simulink model "VCU_SW_1"  (R2023b)
settings: Solver=FixedStepDiscrete  StartTime=0.0  StopTime=inf  FixedStep=1e-2  RelTol=1e-3
PreLoadFcn:
  | RTWConfigurationCB('preloadfcn', bdroot);
InitFcn:
  | loadvar_ttc500
undefined symbols (not defined in the file): BrkPedalTypes, CabMovModeTypes, cFuseTempSensAcc_X, cFuseTempSensAcc_Y, cFuseTempSensVal_X, cFuseTempSensVal_Y, cTMSTempSensVal_X, cTMSTempSensVal_Y, cTransferCaseSpeedRatio, diag_state, DoorsPositionTypes, dP_filter_Y, DriverOccClassSystemTypes, ErrorValueTypes, fatal_error_callback, IO_ADC_NO_RANGE, LadderStatusTypes, pAnalogCabRotSensAcc, pAnalogCabRotSensMaxVolt, pAnalogCabRotSensMinVolt, pAnalogCabRotSensRange, pAnalogCabRotSensZeroVolt, pBrkActivePress, pCabTiltSensAcc, pCabTiltSensMaxCur, pCabTiltSensMinCur, pDistanceCorrection, pECANManual_BPNEnable, pECANManual_BPNEnabler_Flag, pFilterSensAccRes, pHDirMaxDiffFrq, pHDirSensHighLvl, pHDirSensLowLvl, pMainGearRatio, pMaxFilterSensRes, pMaxFirstPedalSensValue, pMaxFuseTempSensRes, pMaxPressLoss, pMaxPressSensCurrent, pMaxPressValue, pMaxPressValueHydMotAndPump, pMaxPressValueParkDrain, pMaxSecondPedalSensValue, pMaxTempSensVoltage, pMaxTempValue, pMaxTMSTempSensRes, pMinFilterSensRes, pMinFirstPedalSensValue, pMinFuseTempSensRes, pMinPressLoss, pMinPressSensCurrent, pMinPressValue, pMinSecondPedalSensValue, pMinTempSensVoltage, pMinTempValue, pMinTMSTempSensRes, pMotorRingTeethNum, pPedalSensAccuracyPct, pPedalSensAccuracyVolt, pPressLossTreshhold ... (+20)
libraries: TTlibrary x270, canmsglib x127, simulink x88
(part 7 of 19)

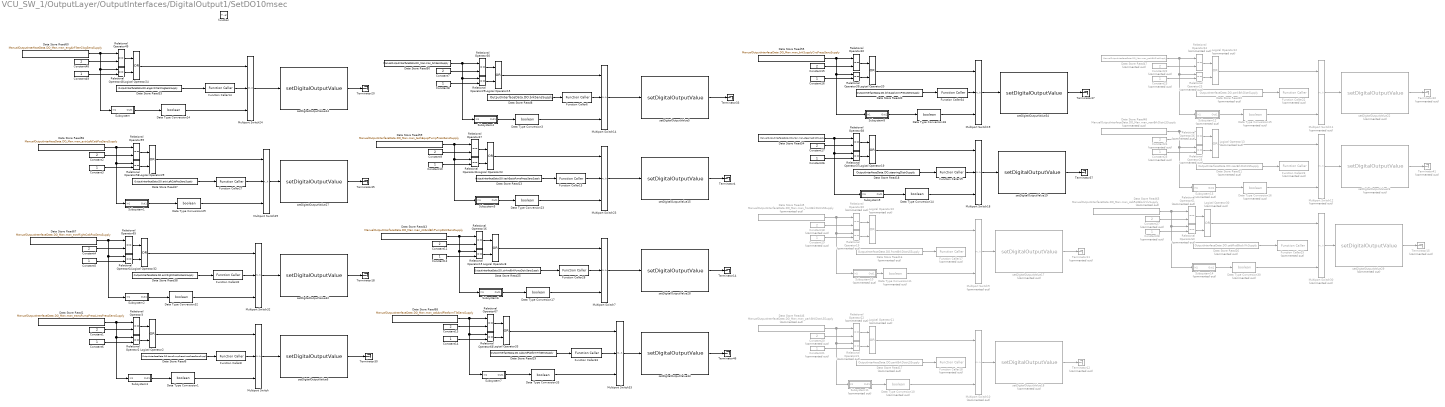
== system VCU_SW_1/OutputLayer/OutputInterfaces/DigitalOutput1/SetDO10msec ==
  function : TriggerPort  TriggerType=function-call  VariantControl=Variant
  Constant{1..2,4,7,9,11,13,15,17,48} (10 alike) : Constant  Value=2  OutDataTypeStr=uint8
  Constant{3,5..6,8,10,12,14,16,26,49} (10 alike) : Constant  OutDataTypeStr=uint8
  Constant{18,20,22,24,27} (5 alike) : Constant  Commented=on  Value=2  OutDataTypeStr=uint8
  Constant{19,21,23,25,28} (5 alike) : Constant  Commented=on  OutDataTypeStr=uint8
  Data Store Read1 : DataStoreRead  DataStoreName=ManualOutputInterfaceData  DataStoreElements=ManualOutputInterfaceData.DO_Man.man_transPumpPressLinesPressSensSupply  IndexOptions=Index vector (dialog)  Indices=1  OutputSizes=1
  Data Store Read13 : DataStoreRead  DataStoreName=OutputInterfaceData  DataStoreElements=OutputInterfaceData.DO.techEquipPumpPressSensSupply  IndexOptions=Index vector (dialog)  Indices=1  OutputSizes=1
  Data Store Read16 : DataStoreRead  Commented=on  DataStoreName=OutputInterfaceData  DataStoreElements=OutputInterfaceData.DO.frontBrkDistrLSSupply  IndexOptions=Index vector (dialog)  Indices=1  OutputSizes=1
  Data Store Read17 : DataStoreRead  Commented=on  DataStoreName=OutputInterfaceData  DataStoreElements=OutputInterfaceData.DO.parkBrkDistrLSSupply  IndexOptions=Index vector (dialog)  Indices=1  OutputSizes=1
  Data Store Read18 : DataStoreRead  DataStoreName=OutputInterfaceData  DataStoreElements=OutputInterfaceData.DO.steeringDistrSupply  IndexOptions=Index vector (dialog)  Indices=1  OutputSizes=1
  Data Store Read20 : DataStoreRead  Commented=on  DataStoreName=OutputInterfaceData  DataStoreElements=OutputInterfaceData.DO.parkBrkDistrSupply  IndexOptions=Index vector (dialog)  Indices=1  OutputSizes=1
  Data Store Read21 : DataStoreRead  Commented=on  DataStoreName=OutputInterfaceData  DataStoreElements=OutputInterfaceData.DO.rearBrkDistrLSSupply  IndexOptions=Index vector (dialog)  Indices=1  OutputSizes=1
  Data Store Read25 : DataStoreRead  DataStoreName=OutputInterfaceData  DataStoreElements=OutputInterfaceData.DO.strAndBrkPumpDistrSensSupply  IndexOptions=Index vector (dialog)  Indices=1  OutputSizes=1
  Data Store Read26 : DataStoreRead  Commented=on  DataStoreName=OutputInterfaceData  DataStoreElements=OutputInterfaceData.DO.cabRotBlockVlvSupply  IndexOptions=Index vector (dialog)  Indices=1  OutputSizes=1
  Data Store Read29 : DataStoreRead  DataStoreName=OutputInterfaceData  DataStoreElements=OutputInterfaceData.DO.cabAndPlatformTiltSensSupply  IndexOptions=Index vector (dialog)  Indices=1  OutputSizes=1
  Data Store Read30 : DataStoreRead  DataStoreName=OutputInterfaceData  DataStoreElements=OutputInterfaceData.DO.brkSupplyCircPressSensSupply  IndexOptions=Index vector (dialog)  Indices=1  OutputSizes=1
  Data Store Read33 : DataStoreRead  DataStoreName=OutputInterfaceData  DataStoreElements=OutputInterfaceData.DO.engAirFilterClogSensSupply  IndexOptions=Index vector (dialog)  Indices=1  OutputSizes=1
  Data Store Read37 : DataStoreRead  DataStoreName=OutputInterfaceData  DataStoreElements=OutputInterfaceData.DO.extrLeftCabPosSensSupply  IndexOptions=Index vector (dialog)  Indices=1  OutputSizes=1
  Data Store Read38 : DataStoreRead  DataStoreName=OutputInterfaceData  DataStoreElements=OutputInterfaceData.DO.extrRightCabPosSensSupply  IndexOptions=Index vector (dialog)  Indices=1  OutputSizes=1
  Data Store Read43 : DataStoreRead  DataStoreName=ManualOutputInterfaceData  DataStoreElements=ManualOutputInterfaceData.DO_Man.man_strAndBrkPumpDistrSensSupply  IndexOptions=Index vector (dialog)  Indices=1  OutputSizes=1
  Data Store Read45 : DataStoreRead  Commented=on  DataStoreName=ManualOutputInterfaceData  DataStoreElements=ManualOutputInterfaceData.DO_Man.man_frontBrkDistrLSSupply  IndexOptions=Index vector (dialog)  Indices=1  OutputSizes=1
  Data Store Read46 : DataStoreRead  Commented=on  DataStoreName=ManualOutputInterfaceData  DataStoreElements=ManualOutputInterfaceData.DO_Man.man_parkBrkDistrLSSupply  IndexOptions=Index vector (dialog)  Indices=1  OutputSizes=1
  Data Store Read47 : DataStoreRead  Commented=on  DataStoreName=ManualOutputInterfaceData  DataStoreElements=ManualOutputInterfaceData.DO_Man.man_parkBrkDistrSupply  IndexOptions=Index vector (dialog)  Indices=1  OutputSizes=1
  Data Store Read48 : DataStoreRead  Commented=on  DataStoreName=ManualOutputInterfaceData  DataStoreElements=ManualOutputInterfaceData.DO_Man.man_rearBrkDistrLSSupply  IndexOptions=Index vector (dialog)  Indices=1  OutputSizes=1
  Data Store Read50 : DataStoreRead  DataStoreName=ManualOutputInterfaceData  DataStoreElements=ManualOutputInterfaceData.DO_Man.man_brkSensSupply  IndexOptions=Index vector (dialog)  Indices=1  OutputSizes=1
  Data Store Read54 : DataStoreRead  DataStoreName=ManualOutputInterfaceData  DataStoreElements=ManualOutputInterfaceData.DO_Man.man_steeringDistrSupply  IndexOptions=Index vector (dialog)  Indices=1  OutputSizes=1
  Data Store Read55 : DataStoreRead  DataStoreName=ManualOutputInterfaceData  DataStoreElements=ManualOutputInterfaceData.DO_Man.man_brkSupplyCircPressSensSupply  IndexOptions=Index vector (dialog)  Indices=1  OutputSizes=1
  Data Store Read58 : DataStoreRead  DataStoreName=ManualOutputInterfaceData  DataStoreElements=ManualOutputInterfaceData.DO_Man.man_extrLeftCabPosSensSupply  IndexOptions=Index vector (dialog)  Indices=1  OutputSizes=1
  Data Store Read59 : DataStoreRead  DataStoreName=ManualOutputInterfaceData  DataStoreElements=ManualOutputInterfaceData.DO_Man.man_techEquipPumpPressSensSupply  IndexOptions=Index vector (dialog)  Indices=1  OutputSizes=1
  Data Store Read6 : DataStoreRead  DataStoreName=OutputInterfaceData  DataStoreElements=OutputInterfaceData.DO.transPumpPressLinesPressSensSupply  IndexOptions=Index vector (dialog)  Indices=1  OutputSizes=1
  Data Store Read60 : DataStoreRead  DataStoreName=ManualOutputInterfaceData  DataStoreElements=ManualOutputInterfaceData.DO_Man.man_engAirFilterClogSensSupply  IndexOptions=Index vector (dialog)  Indices=1  OutputSizes=1
  Data Store Read65 : DataStoreRead  Commented=on  DataStoreName=ManualOutputInterfaceData  DataStoreElements=ManualOutputInterfaceData.DO_Man.man_cabRotBlockVlvSupply  IndexOptions=Index vector (dialog)  Indices=1  OutputSizes=1
  Data Store Read67 : DataStoreRead  DataStoreName=ManualOutputInterfaceData  DataStoreElements=ManualOutputInterfaceData.DO_Man.man_extrRightCabPosSensSupply  IndexOptions=Index vector (dialog)  Indices=1  OutputSizes=1
  Data Store Read68 : DataStoreRead  DataStoreName=ManualOutputInterfaceData  DataStoreElements=ManualOutputInterfaceData.DO_Man.man_cabAndPlatformTiltSensSupply  IndexOptions=Index vector (dialog)  Indices=1  OutputSizes=1
  Data Store Read8 : DataStoreRead  DataStoreName=OutputInterfaceData  DataStoreElements=OutputInterfaceData.DO.brkSensSupply  IndexOptions=Index vector (dialog)  Indices=1  OutputSizes=1
  Data Type Conversion{1,3,14,17..18,23..24,29,32..33} (10 alike) : DataTypeConversion  OutDataTypeStr=boolean  SaturateOnIntegerOverflow=off  RndMeth=Floor
  Data Type Conversion{10..11,15..16,30} (5 alike) : DataTypeConversion  Commented=on  OutDataTypeStr=boolean  SaturateOnIntegerOverflow=off  RndMeth=Floor
  Function Caller{6,8,14..15,19,27..28,32..34} (10 alike) : FunctionCaller  FunctionPrototype=rawValue = convDIOStsTypeToNum(enumValue)  InputArgumentSpecifications=<Enter example>  OutputArgumentSpecifications=<Enter example>
  Function Caller{17..18,22..23,25} (5 alike) : FunctionCaller  Commented=on  FunctionPrototype=rawValue = convDIOStsTypeToNum(enumValue)  InputArgumentSpecifications=<Enter example>  OutputArgumentSpecifications=<Enter example>
  Logical Operator{10..13,30} (5 alike) : Logic  Commented=on  Operator=OR  AllPortsSameDT=off  OutDataTypeStr=boolean
  Logical Operator{2,8,15,19..20,23..24,29,32..33} (10 alike) : Logic  Operator=OR  AllPortsSameDT=off  OutDataTypeStr=boolean
  Multiport Switch{,7,14,18..19,23..24,29,32..33} (10 alike) : MultiPortSwitch  DataPortOrder=Zero-based contiguous  Inputs=2  zeroidx=on  SaturateOnIntegerOverflow=off  InputSameDT=off
  Multiport Switch{9..12,30} (5 alike) : MultiPortSwitch  Commented=on  DataPortOrder=Zero-based contiguous  Inputs=2  zeroidx=on  SaturateOnIntegerOverflow=off  InputSameDT=off
  Relational Operator{2..3,15..16,29..30,37..40,46..49,58..59,64..67} (20 alike) : RelationalOperator  Operator===  OutDataTypeStr=boolean  RndMeth=Simplest  InputSameDT=off
  Relational Operator{19..26,60..61} (10 alike) : RelationalOperator  Commented=on  Operator===  OutDataTypeStr=boolean  RndMeth=Simplest  InputSameDT=off
  Subsystem : Subsystem
  Subsystem1 : Subsystem
  Subsystem10 : Subsystem  Commented=on
  Subsystem11 : Subsystem  Commented=on
  Subsystem12 : Subsystem  Commented=on
  Subsystem13 : Subsystem  Commented=on
  Subsystem14 : Subsystem  Commented=on
  Subsystem2 : Subsystem
  Subsystem3 : Subsystem
  Subsystem4 : Subsystem
  Subsystem5 : Subsystem
  Subsystem6 : Subsystem
  Subsystem7 : Subsystem
  Subsystem8 : Subsystem
  Subsystem9 : Subsystem
  Terminator{11..12,15,40..41} (5 alike) : Terminator  Commented=on
  Terminator{4,14,18,20,30,33,37,45..47} (10 alike) : Terminator
  setDigitalOutputValue14 : TTlibrary/DIO/setDigitalOutputValue  do_channel=IO_DO_55  diagnostic=FALSE  safety_conf=off  low_side_safety_channel=IO_DO_08  io_error=on  sample_time=-1
      settings: SourceProductName=TT control 500 series
  setDigitalOutputValue15 : TTlibrary/DIO/setDigitalOutputValue  do_channel=IO_DO_27  diagnostic=FALSE  safety_conf=off  low_side_safety_channel=IO_DO_08  io_error=on  sample_time=-1
      settings: SourceProductName=TT control 500 series
  setDigitalOutputValue17 : TTlibrary/DIO/setDigitalOutputValue  Commented=on  do_channel=IO_DO_29  diagnostic=FALSE  safety_conf=off  low_side_safety_channel=IO_DO_08  io_error=on  sample_time=-1
      settings: SourceProductName=TT control 500 series
  setDigitalOutputValue18 : TTlibrary/DIO/setDigitalOutputValue  Commented=on  do_channel=IO_DO_43  diagnostic=FALSE  safety_conf=off  low_side_safety_channel=IO_DO_08  io_error=on  sample_time=-1
      settings: SourceProductName=TT control 500 series
  setDigitalOutputValue19 : TTlibrary/DIO/setDigitalOutputValue  do_channel=IO_DO_47  diagnostic=FALSE  safety_conf=off  low_side_safety_channel=IO_DO_08  io_error=on  sample_time=-1
      settings: SourceProductName=TT control 500 series
  setDigitalOutputValue22 : TTlibrary/DIO/setDigitalOutputValue  Commented=on  do_channel=IO_DO_17  diagnostic=FALSE  safety_conf=off  low_side_safety_channel=IO_DO_08  io_error=on  sample_time=-1
      settings: SourceProductName=TT control 500 series
  setDigitalOutputValue23 : TTlibrary/DIO/setDigitalOutputValue  Commented=on  do_channel=IO_DO_31  diagnostic=FALSE  safety_conf=off  low_side_safety_channel=IO_DO_08  io_error=on  sample_time=-1
      settings: SourceProductName=TT control 500 series
  setDigitalOutputValue27 : TTlibrary/DIO/setDigitalOutputValue  do_channel=IO_DO_53  diagnostic=FALSE  safety_conf=off  low_side_safety_channel=IO_DO_08  io_error=on  sample_time=-1
      settings: SourceProductName=TT control 500 series
  setDigitalOutputValue28 : TTlibrary/DIO/setDigitalOutputValue  do_channel=IO_DO_22  diagnostic=FALSE  safety_conf=off  low_side_safety_channel=IO_DO_08  io_error=on  sample_time=-1
      settings: SourceProductName=TT control 500 series
  setDigitalOutputValue29 : TTlibrary/DIO/setDigitalOutputValue  Commented=on  do_channel=IO_DO_36  diagnostic=FALSE  safety_conf=off  low_side_safety_channel=IO_DO_08  io_error=on  sample_time=-1
      settings: SourceProductName=TT control 500 series
  setDigitalOutputValue32 : TTlibrary/DIO/setDigitalOutputValue  do_channel=IO_DO_56  diagnostic=FALSE  safety_conf=off  low_side_safety_channel=IO_DO_08  io_error=on  sample_time=-1
      settings: SourceProductName=TT control 500 series
  setDigitalOutputValue33 : TTlibrary/DIO/setDigitalOutputValue  do_channel=IO_DO_26  diagnostic=FALSE  safety_conf=off  low_side_safety_channel=IO_DO_08  io_error=on  sample_time=-1
      settings: SourceProductName=TT control 500 series
  setDigitalOutputValue34 : TTlibrary/DIO/setDigitalOutputValue  do_channel=IO_DO_40  diagnostic=FALSE  safety_conf=off  low_side_safety_channel=IO_DO_08  io_error=on  sample_time=-1
      settings: SourceProductName=TT control 500 series
  setDigitalOutputValue5 : TTlibrary/DIO/setDigitalOutputValue  do_channel=IO_DO_16  diagnostic=FALSE  safety_conf=off  low_side_safety_channel=IO_DO_08  io_error=on  sample_time=-1
      settings: SourceProductName=TT control 500 series
  setDigitalOutputValue6 : TTlibrary/DIO/setDigitalOutputValue  do_channel=IO_DO_46  diagnostic=FALSE  safety_conf=off  low_side_safety_channel=IO_DO_08  io_error=on  sample_time=-1
      settings: SourceProductName=TT control 500 series
  wires:
  Multiport Switch24/1 -> setDigitalOutputValue14/1
  Function Caller14/1 -> Multiport Switch24/2
  Relational Operator48/1 -> Logical Operator24/2
  Logical Operator24/1 -> Multiport Switch24/1
  Constant48/1 -> Relational Operator49/2
  Data Store Read60/1 -> Relational Operator49/1, Relational Operator48/1, Subsystem/1(In1)
  Relational Operator49/1 -> Logical Operator24/1
  Constant49/1 -> Relational Operator48/2
  Data Type Conversion24/1 -> Multiport Switch24/3
  Data Store Read33/1 -> Function Caller14/1
  setDigitalOutputValue14/1 -> Terminator20/1
  Data Store Read58/1 -> Relational Operator59/1, Relational Operator58/1, Subsystem1/1(In1)
  Relational Operator58/1 -> Logical Operator29/2
  Multiport Switch29/1 -> setDigitalOutputValue27/1
  Relational Operator59/1 -> Logical Operator29/1
  Data Store Read37/1 -> Function Caller27/1
  setDigitalOutputValue27/1 -> Terminator45/1
  Constant2/1 -> Relational Operator59/2
  Function Caller27/1 -> Multiport Switch29/2
  Constant3/1 -> Relational Operator58/2
  Data Type Conversion29/1 -> Multiport Switch29/3
  Logical Operator29/1 -> Multiport Switch29/1
  Logical Operator32/1 -> Multiport Switch32/1
  Function Caller32/1 -> Multiport Switch32/2
  setDigitalOutputValue32/1 -> Terminator18/1
  Data Store Read38/1 -> Function Caller32/1
  Data Store Read67/1 -> Relational Operator65/1, Relational Operator64/1, Subsystem2/1(In1)
  Constant5/1 -> Relational Operator64/2
  Relational Operator64/1 -> Logical Operator32/2
  Multiport Switch32/1 -> setDigitalOutputValue32/1
  Data Type Conversion32/1 -> Multiport Switch32/3
  Relational Operator65/1 -> Logical Operator32/1
  Constant4/1 -> Relational Operator65/2
  Logical Operator2/1 -> Multiport Switch/1
  Multiport Switch/1 -> setDigitalOutputValue6/1
  Relational Operator3/1 -> Logical Operator2/1
  Data Store Read1/1 -> Relational Operator3/1, Relational Operator2/1, Subsystem3/1(In1)
  Data Type Conversion1/1 -> Multiport Switch/3
  Relational Operator2/1 -> Logical Operator2/2
  Constant1/1 -> Relational Operator3/2
  Data Store Read6/1 -> Function Caller8/1
  setDigitalOutputValue6/1 -> Terminator30/1
  Function Caller8/1 -> Multiport Switch/2
  Constant6/1 -> Relational Operator2/2
  Data Store Read13/1 -> Function Caller15/1
  Constant10/1 -> Relational Operator46/2
  Function Caller15/1 -> Multiport Switch23/2
  Logical Operator23/1 -> Multiport Switch23/1
  Data Type Conversion23/1 -> Multiport Switch23/3
  Data Store Read59/1 -> Relational Operator47/1, Relational Operator46/1, Subsystem5/1(In1)
  Relational Operator47/1 -> Logical Operator23/1
  Relational Operator46/1 -> Logical Operator23/2
  Multiport Switch23/1 -> setDigitalOutputValue15/1
  setDigitalOutputValue15/1 -> Terminator4/1
  Constant9/1 -> Relational Operator47/2
  Data Type Conversion17/1 -> Multiport Switch7/3
  Constant11/1 -> Relational Operator16/2
  Data Store Read25/1 -> Function Caller28/1
  Multiport Switch7/1 -> setDigitalOutputValue28/1
  Function Caller28/1 -> Multiport Switch7/2
  Data Store Read43/1 -> Relational Operator16/1, Relational Operator15/1, Subsystem6/1(In1)
  setDigitalOutputValue28/1 -> Terminator14/1
  Logical Operator8/1 -> Multiport Switch7/1
  Relational Operator15/1 -> Logical Operator8/2
  Constant12/1 -> Relational Operator15/2
  Relational Operator16/1 -> Logical Operator8/1
  Relational Operator39/1 -> Logical Operator20/2
  Relational Operator67/1 -> Logical Operator33/1
  Multiport Switch33/1 -> setDigitalOutputValue33/1
  Relational Operator40/1 -> Logical Operator20/1
  Logical Operator33/1 -> Multiport Switch33/1
  Relational Operator66/1 -> Logical Operator33/2
  Data Store Read68/1 -> Relational Operator67/1, Relational Operator66/1, Subsystem7/1(In1)
  Logical Operator20/1 -> Multiport Switch19/1
  Data Type Conversion33/1 -> Multiport Switch33/3
  setDigitalOutputValue33/1 -> Terminator46/1
  Constant15/1 -> Relational Operator40/2
  Constant13/1 -> Relational Operator67/2
  Data Store Read55/1 -> Relational Operator40/1, Relational Operator39/1, Subsystem8/1(In1)
  Constant16/1 -> Relational Operator39/2
  Multiport Switch19/1 -> setDigitalOutputValue34/1
  Data Store Read29/1 -> Function Caller33/1
  Function Caller33/1 -> Multiport Switch33/2
  Constant14/1 -> Relational Operator66/2
  Data Store Read30/1 -> Function Caller34/1
  Data Type Conversion18/1 -> Multiport Switch19/3
  setDigitalOutputValue34/1 -> Terminator47/1
  Function Caller34/1 -> Multiport Switch19/2
  Relational Operator37/1 -> Logical Operator19/2
  Logical Operator19/1 -> Multiport Switch18/1
  Constant26/1 -> Relational Operator37/2
  Data Type Conversion14/1 -> Multiport Switch18/3
  setDigitalOutputValue19/1 -> Terminator37/1
  Constant17/1 -> Relational Operator38/2
  Multiport Switch18/1 -> setDigitalOutputValue19/1
  Data Store Read18/1 -> Function Caller19/1
  Relational Operator38/1 -> Logical Operator19/1
  Data Store Read54/1 -> Relational Operator38/1, Relational Operator37/1, Subsystem9/1(In1)
  Function Caller19/1 -> Multiport Switch18/2
  Data Type Conversion3/1 -> Multiport Switch14/3
  Multiport Switch14/1 -> setDigitalOutputValue5/1
  Constant7/1 -> Relational Operator30/2
  Constant8/1 -> Relational Operator29/2
  Logical Operator15/1 -> Multiport Switch14/1
  Data Store Read50/1 -> Relational Operator30/1, Relational Operator29/1, Subsystem4/1(In1)
  Data Store Read8/1 -> Function Caller6/1
  setDigitalOutputValue5/1 -> Terminator33/1
  Relational Operator29/1 -> Logical Operator15/2
  Relational Operator30/1 -> Logical Operator15/1
  Function Caller6/1 -> Multiport Switch14/2
  Relational Operator19/1 -> Logical Operator10/2
  Logical Operator10/1 -> Multiport Switch9/1
  setDigitalOutputValue17/1 -> Terminator11/1
  Constant20/1 -> Relational Operator22/2
  Data Store Read17/1 -> Function Caller18/1
  Relational Operator21/1 -> Logical Operator11/2
  setDigitalOutputValue18/1 -> Terminator12/1
  Multiport Switch9/1 -> setDigitalOutputValue17/1
  Relational Operator22/1 -> Logical Operator11/1
  Data Store Read16/1 -> Function Caller17/1
  Constant19/1 -> Relational Operator19/2
  Logical Operator11/1 -> Multiport Switch10/1
  Constant21/1 -> Relational Operator21/2
  Multiport Switch10/1 -> setDigitalOutputValue18/1
  Relational Operator20/1 -> Logical Operator10/1
  Data Type Conversion10/1 -> Multiport Switch10/3
  Data Type Conversion11/1 -> Multiport Switch9/3
  Constant18/1 -> Relational Operator20/2
  Data Store Read45/1 -> Relational Operator20/1, Relational Operator19/1, Subsystem10/1(In1)
  Data Store Read46/1 -> Relational Operator22/1, Relational Operator21/1, Subsystem11/1(In1)
  Constant22/1 -> Relational Operator24/2
  Constant23/1 -> Relational Operator23/2
  Multiport Switch12/1 -> setDigitalOutputValue23/1
  Data Store Read47/1 -> Relational Operator24/1, Relational Operator23/1, Subsystem12/1(In1)
  Relational Operator24/1 -> Logical Operator12/1
  Data Type Conversion15/1 -> Multiport Switch11/3
  Data Store Read21/1 -> Function Caller23/1
  Multiport Switch11/1 -> setDigitalOutputValue22/1
  setDigitalOutputValue23/1 -> Terminator41/1
  Constant25/1 -> Relational Operator25/2
  Data Type Conversion16/1 -> Multiport Switch12/3
  Logical Operator13/1 -> Multiport Switch12/1
  Data Store Read48/1 -> Relational Operator26/1, Relational Operator25/1, Subsystem13/1(In1)
  Relational Operator25/1 -> Logical Operator13/2
  Constant24/1 -> Relational Operator26/2
  Relational Operator23/1 -> Logical Operator12/2
  Relational Operator26/1 -> Logical Operator13/1
  Logical Operator12/1 -> Multiport Switch11/1
  setDigitalOutputValue22/1 -> Terminator40/1
  Data Store Read20/1 -> Function Caller22/1
  Data Store Read65/1 -> Relational Operator61/1, Relational Operator60/1, Subsystem14/1(In1)
  setDigitalOutputValue29/1 -> Terminator15/1
  Logical Operator30/1 -> Multiport Switch30/1
  Constant27/1 -> Relational Operator61/2
  Relational Operator60/1 -> Logical Operator30/2
  Data Store Read26/1 -> Function Caller25/1
  Multiport Switch30/1 -> setDigitalOutputValue29/1
  Constant28/1 -> Relational Operator60/2
  Data Type Conversion30/1 -> Multiport Switch30/3
  Relational Operator61/1 -> Logical Operator30/1
  Subsystem/1(Out1) -> Data Type Conversion24/1
  Subsystem1/1(Out1) -> Data Type Conversion29/1
  Subsystem2/1(Out1) -> Data Type Conversion32/1
  Subsystem3/1(Out1) -> Data Type Conversion1/1
  Subsystem4/1(Out1) -> Data Type Conversion3/1
  Subsystem5/1(Out1) -> Data Type Conversion23/1
  Subsystem6/1(Out1) -> Data Type Conversion17/1
  Subsystem7/1(Out1) -> Data Type Conversion33/1
  Subsystem8/1(Out1) -> Data Type Conversion18/1
  Subsystem9/1(Out1) -> Data Type Conversion14/1
  Subsystem10/1(Out1) -> Data Type Conversion11/1
  Subsystem11/1(Out1) -> Data Type Conversion10/1
  Subsystem12/1(Out1) -> Data Type Conversion15/1
  Subsystem13/1(Out1) -> Data Type Conversion16/1
  Subsystem14/1(Out1) -> Data Type Conversion30/1

== system VCU_SW_1/OutputLayer/OutputInterfaces/PWMOutput/SetPWM1000msec ==
  function : TriggerPort  TriggerType=function-call  VariantControl=Variant

== system VCU_SW_1/OutputLayer/OutputInterfaces/PWMOutput/SetPWM10msec ==
  function : TriggerPort  TriggerType=function-call  VariantControl=Variant
  Data Store Read1 : DataStoreRead  DataStoreName=OutputInterfaceData  DataStoreElements=OutputInterfaceData.PWM.driveTransPumpVlv  IndexOptions=Index vector (dialog)  Indices=1  OutputSizes=1
  Data Store Read2 : DataStoreRead  DataStoreName=OutputInterfaceData  DataStoreElements=OutputInterfaceData.PWM.reverseTransPumpVlv  IndexOptions=Index vector (dialog)  Indices=1  OutputSizes=1
  Data Store Read22 : DataStoreRead  Commented=on  DataStoreName=OutputInterfaceData  DataStoreElements=OutputInterfaceData.PWM.spareBrkDistrSupply  IndexOptions=Index vector (dialog)  Indices=1  OutputSizes=1
  Data Store Read3 : DataStoreRead  DataStoreName=OutputInterfaceData  DataStoreElements=OutputInterfaceData.PWM.transPumpVlv  IndexOptions=Index vector (dialog)  Indices=1  OutputSizes=1
  Data Store Read36 : DataStoreRead  DataStoreName=OutputInterfaceData  DataStoreElements=OutputInterfaceData.PWM.strAndBrkPumpDistrSupply  IndexOptions=Index vector (dialog)  Indices=1  OutputSizes=1
  Data Store Read4 : DataStoreRead  DataStoreName=OutputInterfaceData  DataStoreElements=OutputInterfaceData.PWM.techEquipPumpSupply  IndexOptions=Index vector (dialog)  Indices=1  OutputSizes=1
  Terminator{1..4,13} (5 alike) : Terminator
  Terminator21 : Terminator  Commented=on
  pwmSetDutyCycle1 : TTlibrary/PWM /pwmSetDutyCycle  pwm_channel=IO_PWM_19  frequency=1000  polarity=TRUE  diag_margin=FALSE  activate_feedback=off  safety_conf=off  init_with_low_side=on  enable_current_check=TRUE  current_limit=2000  low_side_channel=IO_DO_08  io_error=on  sample_time=-1
      settings: SourceProductName=TT control 500 series
  pwmSetDutyCycle2 : TTlibrary/PWM /pwmSetDutyCycle  pwm_channel=IO_PWM_28  frequency=100  polarity=TRUE  diag_margin=FALSE  activate_feedback=off  safety_conf=off  init_with_low_side=on  enable_current_check=TRUE  current_limit=2000  low_side_channel=IO_DO_08  io_error=on  sample_time=-1
      settings: SourceProductName=TT control 500 series
  pwmSetDutyCycle21 : TTlibrary/PWM /pwmSetDutyCycle  Commented=on  pwm_channel=IO_PWM_03  frequency=1000  polarity=TRUE  diag_margin=FALSE  activate_feedback=off  safety_conf=off  init_with_low_side=on  enable_current_check=TRUE  current_limit=2000  low_side_channel=IO_DO_08  io_error=on  sample_time=-1
      settings: SourceProductName=TT control 500 series
  pwmSetDutyCycle3 : TTlibrary/PWM /pwmSetDutyCycle  pwm_channel=IO_PWM_32  frequency=100  polarity=TRUE  diag_margin=FALSE  activate_feedback=off  safety_conf=off  init_with_low_side=on  enable_current_check=TRUE  current_limit=2000  low_side_channel=IO_DO_08  io_error=on  sample_time=-1
      settings: SourceProductName=TT control 500 series
  pwmSetDutyCycle4 : TTlibrary/PWM /pwmSetDutyCycle  pwm_channel=IO_PWM_33  frequency=100  polarity=TRUE  diag_margin=FALSE  activate_feedback=off  safety_conf=off  init_with_low_side=on  enable_current_check=TRUE  current_limit=2000  low_side_channel=IO_DO_08  io_error=on  sample_time=-1
      settings: SourceProductName=TT control 500 series
  pwmSetDutyCycle5 : TTlibrary/PWM /pwmSetDutyCycle  pwm_channel=IO_PWM_14  frequency=1000  polarity=TRUE  diag_margin=FALSE  activate_feedback=off  safety_conf=off  init_with_low_side=on  enable_current_check=TRUE  current_limit=2000  low_side_channel=IO_DO_08  io_error=on  sample_time=-1
      settings: SourceProductName=TT control 500 series
  wires:
  pwmSetDutyCycle21/1 -> Terminator21/1  "io_pwm_03_error"
  pwmSetDutyCycle1/1 -> Terminator13/1  "io_pwm_19_error"
  pwmSetDutyCycle2/1 -> Terminator1/1  "io_pwm_28_error"
  pwmSetDutyCycle3/1 -> Terminator2/1  "io_pwm_32_error"
  pwmSetDutyCycle4/1 -> Terminator3/1  "io_pwm_33_error"
  Data Store Read3/1 -> pwmSetDutyCycle4/1
  pwmSetDutyCycle5/1 -> Terminator4/1  "io_pwm_14_error"
  Data Store Read4/1 -> pwmSetDutyCycle5/1
  Data Store Read1/1 -> pwmSetDutyCycle2/1
  Data Store Read2/1 -> pwmSetDutyCycle3/1
  Data Store Read22/1 -> pwmSetDutyCycle21/1
  Data Store Read36/1 -> pwmSetDutyCycle1/1

== system VCU_SW_1/OutputLayer/OutputInterfaces/exDigitalOutput/SetDO1000msec ==
  function : TriggerPort  TriggerType=function-call  VariantControl=Variant
  Constant50 : Constant  OutDataTypeStr=uint8
  Constant51 : Constant  Value=0  OutDataTypeStr=uint8
  Data Store Read15 : DataStoreRead  DataStoreName=OutputInterfaceData  DataStoreElements=OutputInterfaceData.DO.lowBrakeFluidSensSupply  IndexOptions=Index vector (dialog)  Indices=1  OutputSizes=1
  Data Store Read61 : DataStoreRead  DataStoreName=ManualOutputInterfaceData  DataStoreElements=ManualOutputInterfaceData.DO_Man.man_lowBrakeFluidSensSupply  IndexOptions=Index vector (dialog)  Indices=1  OutputSizes=1
  Data Type Conversion25 : DataTypeConversion  OutDataTypeStr=boolean  SaturateOnIntegerOverflow=off  RndMeth=Floor
  Function Caller16 : FunctionCaller  FunctionPrototype=rawValue = convDIOStsTypeToNum(enumValue)  InputArgumentSpecifications=<Enter example>  OutputArgumentSpecifications=<Enter example>
  Logical Operator25 : Logic  Operator=OR  AllPortsSameDT=off  OutDataTypeStr=boolean
  Multiport Switch25 : MultiPortSwitch  DataPortOrder=Zero-based contiguous  Inputs=2  zeroidx=on  SaturateOnIntegerOverflow=off  InputSameDT=off
  Relational Operator50 : RelationalOperator  Operator===  OutDataTypeStr=boolean  RndMeth=Simplest  InputSameDT=off
  Relational Operator51 : RelationalOperator  Operator===  OutDataTypeStr=boolean  RndMeth=Simplest  InputSameDT=off
  Terminator10 : Terminator
  setDigitalOutputValue16 : TTlibrary/DIO/setDigitalOutputValue  do_channel=IO_DO_41  diagnostic=FALSE  safety_conf=off  low_side_safety_channel=IO_DO_08  io_error=on  sample_time=-1
      settings: SourceProductName=TT control 500 series
  wires:
  Data Type Conversion25/1 -> Multiport Switch25/3
  Constant51/1 -> Relational Operator50/2
  Relational Operator50/1 -> Logical Operator25/2
  Multiport Switch25/1 -> setDigitalOutputValue16/1
  Logical Operator25/1 -> Multiport Switch25/1
  Data Store Read15/1 -> Function Caller16/1
  Relational Operator51/1 -> Logical Operator25/1
  Data Store Read61/1 -> Relational Operator51/1, Relational Operator50/1, Data Type Conversion25/1
  setDigitalOutputValue16/1 -> Terminator10/1
  Constant50/1 -> Relational Operator51/2
  Function Caller16/1 -> Multiport Switch25/2
